simulink model "FFR_3area"  (R2015a)
settings: Solver=ode45  StartTime=0.0  StopTime=20  RelTol=1e-3
values from neighbouring files (symbols this model uses):
  beta = [0.3483 0.3827 0.3692]    [init_FFR_3area.m]    (also in init_FFR_3area_2.m; init_FFR_3area_3.m; init_FFR_3area_4.m; init_FFR_3area_5.m)
  D = 0.015    [init_FFR_1_0.m]    (also in init_FFR_1_1.m; init_FFR_3area.m = [0.015 0.016 0.015]; init_FFR_3area_2.m = [0.015 0.016 0.015]; init_FFR_3area_3.m = [0.015 0.016 0.015])
  H = 0.0833    [init_FFR_1_0.m]    (also in init_FFR_1_1.m; init_FFR_3area.m = [0.1667 0.2017 0.1247] .* 0.5; init_FFR_3area_2.m = [0.1667 0.2017 0.1247] .* 0.5; init_FFR_3area_3.m = [0.1667 0.2017 0.1247] .* 0.5)
  Ki = -0.3    [init_FFR_1_0.m]    (also in init_FFR_1_1.m = -2; init_FFR_3area.m = [-0.3 -0.2 -0.4]; init_FFR_3area_2.m = [-0.3 -0.2 -0.4]; init_FFR_3area_3.m = [-0.3 -0.2 -0.4])
  R = 3    [init_FFR_1_0.m]    (also in init_FFR_1_1.m; init_FFR_3area.m = [3 2.73 2.82]; init_FFR_3area_2.m = [3 2.73 2.82]; init_FFR_3area_3.m = [3 2.73 2.82])
  T_12 = 0.20    (= 0.2)    [allocateProduction.m]    (also in allocation.m; init_FFR_3area.m; init_FFR_3area_2.m; init_FFR_3area_3.m)
  T_13 = 0.25    [allocateProduction.m]    (also in allocation.m; init_FFR_3area.m; init_FFR_3area_2.m; init_FFR_3area_3.m)
  T_21 = 0.20    (= 0.2)    [allocateProduction.m]    (also in allocation.m; init_FFR_3area.m; init_FFR_3area_2.m; init_FFR_3area_3.m)
  T_23 = 0.12    [allocateProduction.m]    (also in allocation.m; init_FFR_3area.m; init_FFR_3area_2.m; init_FFR_3area_3.m)
  T_31 = 0.25    [allocateProduction.m]    (also in allocation.m; init_FFR_3area.m; init_FFR_3area_2.m; init_FFR_3area_3.m)
  T_32 = 0.12    [allocateProduction.m]    (also in allocation.m; init_FFR_3area.m; init_FFR_3area_2.m; init_FFR_3area_3.m)
  T_g = 0.08    [init_FFR_1_0.m]    (also in init_FFR_1_1.m; init_FFR_3area.m = [0.08 0.06 0.07]; init_FFR_3area_2.m = [0.08 0.06 0.07]; init_FFR_3area_3.m = [0.08 0.06 0.07])
  T_t = 0.40    (= 0.4)    [init_FFR_1_0.m]    (also in init_FFR_1_1.m; init_FFR_3area.m = [0.40 0.44 0.30]; init_FFR_3area_2.m = [0.40 0.44 0.30]; init_FFR_3area_3.m = [0.40 0.44 0.30])
settings Model: Creator=tarje  LastModifiedBy=tarje

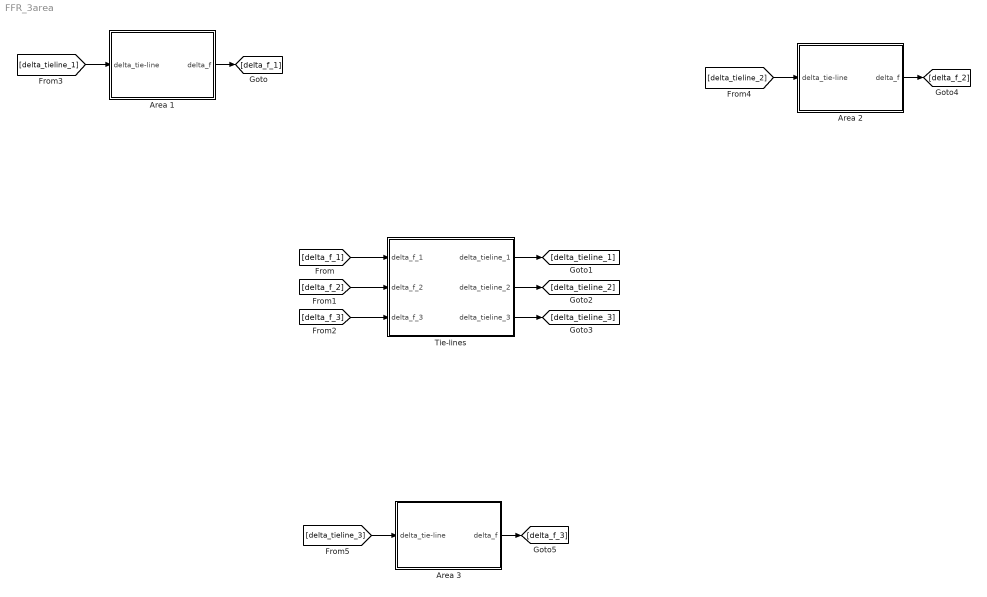
== system FFR_3area ==
  Area 1 : Subsystem
  Area 2 : Subsystem
  Area 3 : Subsystem
  Tie-lines : Subsystem
  wires:
  Area 1/1(delta_f) -> [delta_f_1]
  [delta_f_1] -> Tie-lines/1(delta_f_1)
  Tie-lines/1(delta_tieline_1) -> [delta_tieline_1]
  Tie-lines/2(delta_tieline_2) -> [delta_tieline_2]
  Tie-lines/3(delta_tieline_3) -> [delta_tieline_3]
  [delta_f_2] -> Tie-lines/2(delta_f_2)
  [delta_f_3] -> Tie-lines/3(delta_f_3)
  [delta_tieline_1] -> Area 1/1(delta_tie-line)
  Area 2/1(delta_f) -> [delta_f_2]
  [delta_tieline_2] -> Area 2/1(delta_tie-line)
  Area 3/1(delta_f) -> [delta_f_3]
  [delta_tieline_3] -> Area 3/1(delta_tie-line)

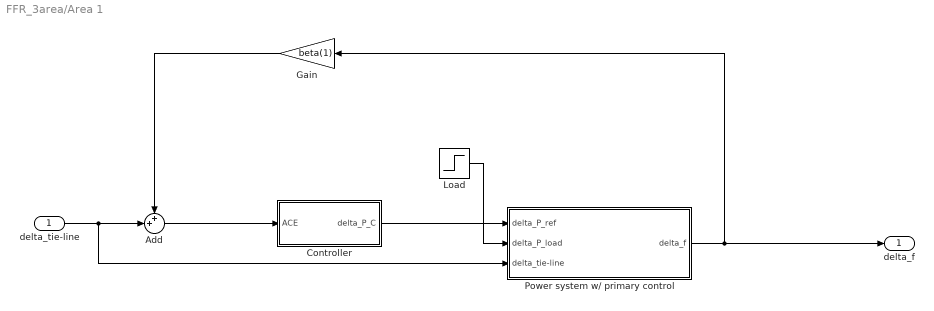
== system FFR_3area/Area 1 ==
  delta_tie-line : Inport
  Add : Sum  Inputs=++|
  Controller : Subsystem
  Gain : Gain  Gain=beta(1)
  Load : Step  Time=2  After=.02  SampleTime=0
  Power system w/ primary control : Subsystem
  delta_f : Outport
  wires:
  Load/1 -> Power system w/ primary control/2(delta_P_load)
  Controller/1(delta_P_C) -> Power system w/ primary control/1(delta_P_ref)
  Power system w/ primary control/1(delta_f) -> Gain/1, delta_f/1
  Gain/1 -> Add/1
  delta_tie-line/1 -> Power system w/ primary control/3(delta_tie-line), Add/2
  Add/1 -> Controller/1(ACE)

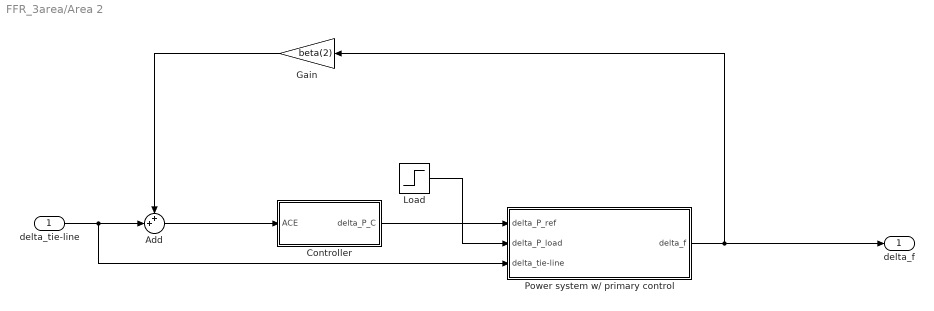
== system FFR_3area/Area 2 ==
  delta_tie-line : Inport
  Add : Sum  Inputs=++|
  Controller : Subsystem
  Gain : Gain  Gain=beta(2)
  Load : Step  Time=2  After=0  SampleTime=0
  Power system w/ primary control : Subsystem
  delta_f : Outport
  wires:
  Load/1 -> Power system w/ primary control/2(delta_P_load)
  Controller/1(delta_P_C) -> Power system w/ primary control/1(delta_P_ref)
  Power system w/ primary control/1(delta_f) -> Gain/1, delta_f/1
  Gain/1 -> Add/1
  delta_tie-line/1 -> Power system w/ primary control/3(delta_tie-line), Add/2
  Add/1 -> Controller/1(ACE)

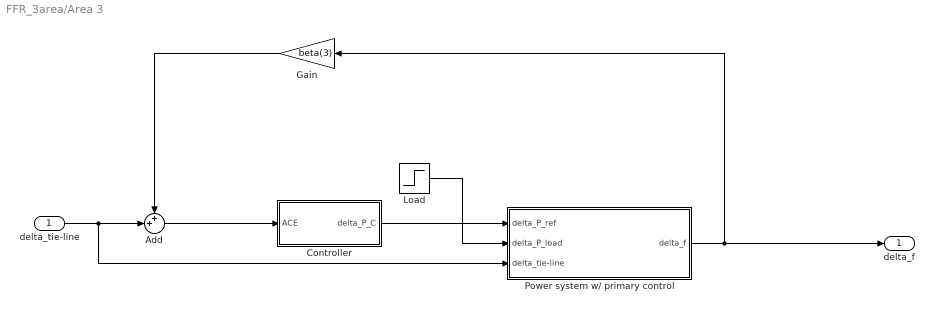
== system FFR_3area/Area 3 ==
  delta_tie-line : Inport
  Add : Sum  Inputs=++|
  Controller : Subsystem
  Gain : Gain  Gain=beta(3)
  Load : Step  Time=2  After=.02  SampleTime=0
  Power system w/ primary control : Subsystem
  delta_f : Outport
  wires:
  Load/1 -> Power system w/ primary control/2(delta_P_load)
  Controller/1(delta_P_C) -> Power system w/ primary control/1(delta_P_ref)
  Power system w/ primary control/1(delta_f) -> Gain/1, delta_f/1
  Gain/1 -> Add/1
  delta_tie-line/1 -> Power system w/ primary control/3(delta_tie-line), Add/2
  Add/1 -> Controller/1(ACE)

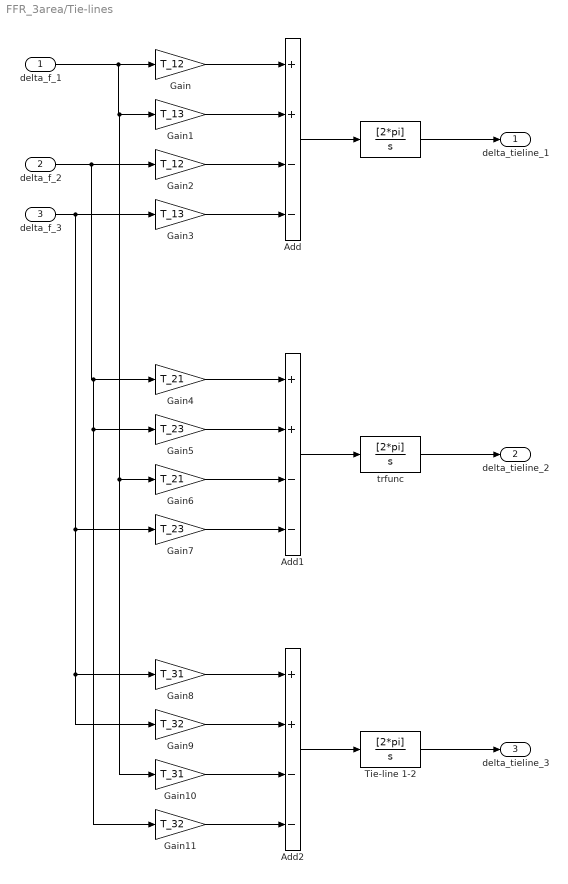
== system FFR_3area/Tie-lines ==
  delta_f_1 : Inport
  delta_f_2 : Inport  Port=2
  delta_f_3 : Inport  Port=3
  " " : TransferFcn  Numerator=[2*pi]  Denominator=[1 0]
  Add : Sum  Inputs=++--
  Add1 : Sum  Inputs=++--
  Add2 : Sum  Inputs=++--
  Gain : Gain  Gain=T_12
  Gain1 : Gain  Gain=T_13
  Gain10 : Gain  Gain=T_31
  Gain11 : Gain  Gain=T_32
  Gain2 : Gain  Gain=T_12
  Gain3 : Gain  Gain=T_13
  Gain4 : Gain  Gain=T_21
  Gain5 : Gain  Gain=T_23
  Gain6 : Gain  Gain=T_21
  Gain7 : Gain  Gain=T_23
  Gain8 : Gain  Gain=T_31
  Gain9 : Gain  Gain=T_32
  Tie-line 1-2 : TransferFcn  Numerator=[2*pi]  Denominator=[1 0]
  trfunc : TransferFcn  Numerator=[2*pi]  Denominator=[1 0]
  delta_tieline_1 : Outport
  delta_tieline_2 : Outport  Port=2
  delta_tieline_3 : Outport  Port=3
  wires:
  Gain/1 -> Add/1
  Gain1/1 -> Add/2
  Gain3/1 -> Add/4
  Gain2/1 -> Add/3
  Add/1 -> " "/1
  " "/1 -> delta_tieline_1/1
  Gain4/1 -> Add1/1
  Gain5/1 -> Add1/2
  Gain7/1 -> Add1/4
  Gain6/1 -> Add1/3
  Add1/1 -> trfunc/1
  trfunc/1 -> delta_tieline_2/1
  delta_f_3/1 -> Gain7/1, Gain9/1, Gain8/1, Gain3/1
  Gain8/1 -> Add2/1
  Gain9/1 -> Add2/2
  Gain11/1 -> Add2/4
  Gain10/1 -> Add2/3
  delta_f_1/1 -> Gain10/1, Gain6/1, Gain1/1, Gain/1
  delta_f_2/1 -> Gain11/1, Gain5/1, Gain4/1, Gain2/1
  Add2/1 -> Tie-line 1-2/1
  Tie-line 1-2/1 -> delta_tieline_3/1

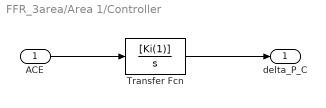
== system FFR_3area/Area 1/Controller ==
  ACE : Inport
  Transfer Fcn : TransferFcn  Numerator=[Ki(1)]  Denominator=[1 0]
  delta_P_C : Outport
  wires:
  ACE/1 -> Transfer Fcn/1
  Transfer Fcn/1 -> delta_P_C/1

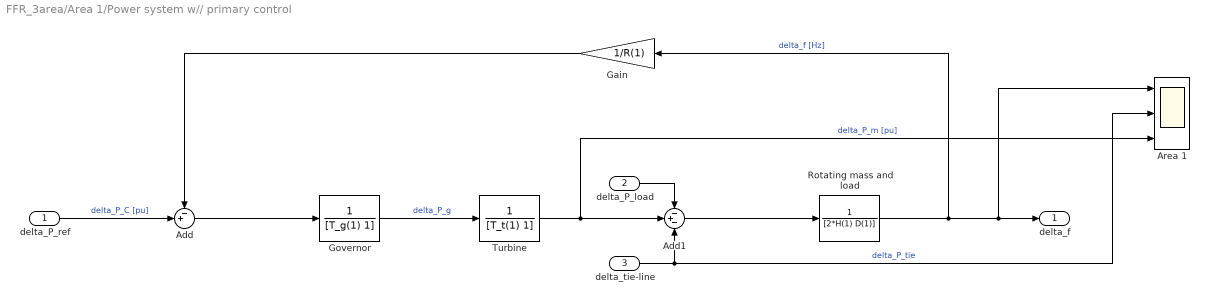
== system FFR_3area/Area 1/Power system w// primary control ==
  delta_P_ref : Inport
  delta_P_load : Inport  Port=2
  delta_tie-line : Inport  Port=3
  Add : Sum  Inputs=-+|
  Add1 : Sum  Inputs=-+-
  Area 1 : Scope  NumInputPorts=3
      settings: TimeRange=3.2  YMin=-0.065~-0.02~-0.01  YMax=0.02~0.025~0.03
  Gain : Gain  Gain=1/R(1)
  Governor : TransferFcn  Denominator=[T_g(1) 1]
  Rotating mass and load : TransferFcn  Denominator=[2*H(1) D(1)]
  Turbine : TransferFcn  Denominator=[T_t(1) 1]
  delta_f : Outport
  wires:
  Turbine/1 -> Area 1/3, Add1/2  "delta_P_m [pu]"
  Rotating mass and load/1 -> Area 1/1, delta_f/1, Gain/1  "delta_f [Hz]"
  Gain/1 -> Add/1
  Add1/1 -> Rotating mass and load/1
  Add/1 -> Governor/1
  Governor/1 -> Turbine/1  "delta_P_g"
  delta_P_ref/1 -> Add/2  "delta_P_C [pu]"
  delta_P_load/1 -> Add1/1
  delta_tie-line/1 -> Area 1/2, Add1/3  "delta_P_tie"

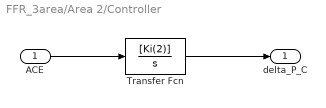
== system FFR_3area/Area 2/Controller ==
  ACE : Inport
  Transfer Fcn : TransferFcn  Numerator=[Ki(2)]  Denominator=[1 0]
  delta_P_C : Outport
  wires:
  ACE/1 -> Transfer Fcn/1
  Transfer Fcn/1 -> delta_P_C/1

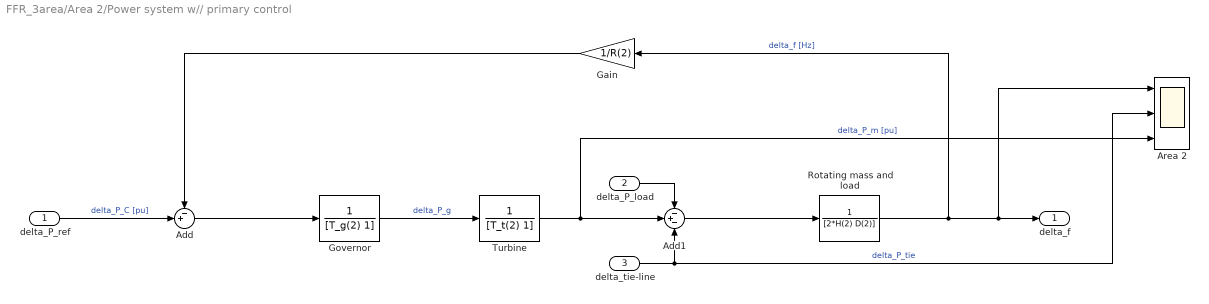
== system FFR_3area/Area 2/Power system w// primary control ==
  delta_P_ref : Inport
  delta_P_load : Inport  Port=2
  delta_tie-line : Inport  Port=3
  Add : Sum  Inputs=-+|
  Add1 : Sum  Inputs=-+-
  Area 2 : Scope  NumInputPorts=3
      settings: TimeRange=15  YMin=-0.08~-0.005~-0.01  YMax=0.025~0.04~0.03
  Gain : Gain  Gain=1/R(2)
  Governor : TransferFcn  Denominator=[T_g(2) 1]
  Rotating mass and load : TransferFcn  Denominator=[2*H(2) D(2)]
  Turbine : TransferFcn  Denominator=[T_t(2) 1]
  delta_f : Outport
  wires:
  Turbine/1 -> Area 2/3, Add1/2  "delta_P_m [pu]"
  Rotating mass and load/1 -> Area 2/1, delta_f/1, Gain/1  "delta_f [Hz]"
  Gain/1 -> Add/1
  Add1/1 -> Rotating mass and load/1
  Add/1 -> Governor/1
  Governor/1 -> Turbine/1  "delta_P_g"
  delta_P_ref/1 -> Add/2  "delta_P_C [pu]"
  delta_P_load/1 -> Add1/1
  delta_tie-line/1 -> Area 2/2, Add1/3  "delta_P_tie"

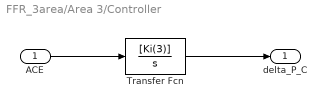
== system FFR_3area/Area 3/Controller ==
  ACE : Inport
  Transfer Fcn : TransferFcn  Numerator=[Ki(3)]  Denominator=[1 0]
  delta_P_C : Outport
  wires:
  ACE/1 -> Transfer Fcn/1
  Transfer Fcn/1 -> delta_P_C/1

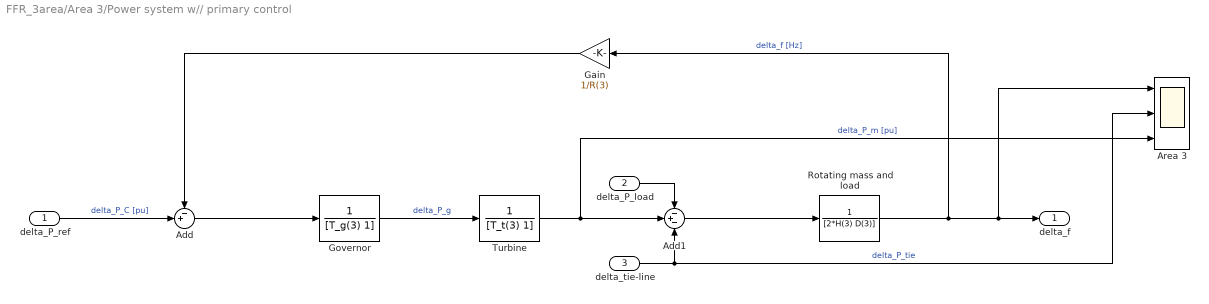
== system FFR_3area/Area 3/Power system w// primary control ==
  delta_P_ref : Inport
  delta_P_load : Inport  Port=2
  delta_tie-line : Inport  Port=3
  Add : Sum  Inputs=-+|
  Add1 : Sum  Inputs=-+-
  Area 3 : Scope  NumInputPorts=3
      settings: TimeRange=15  YMin=-0.08~-0.005~-0.01  YMax=0.025~0.04~0.03
  Gain : Gain  Gain=1/R(3)
  Governor : TransferFcn  Denominator=[T_g(3) 1]
  Rotating mass and load : TransferFcn  Denominator=[2*H(3) D(3)]
  Turbine : TransferFcn  Denominator=[T_t(3) 1]
  delta_f : Outport
  wires:
  Turbine/1 -> Area 3/3, Add1/2  "delta_P_m [pu]"
  Rotating mass and load/1 -> Area 3/1, delta_f/1, Gain/1  "delta_f [Hz]"
  Gain/1 -> Add/1
  Add1/1 -> Rotating mass and load/1
  Add/1 -> Governor/1
  Governor/1 -> Turbine/1  "delta_P_g"
  delta_P_ref/1 -> Add/2  "delta_P_C [pu]"
  delta_P_load/1 -> Add1/1
  delta_tie-line/1 -> Area 3/2, Add1/3  "delta_P_tie"
